simulink model "my_fuzzy"  (Simulink 7.3)
settings: Solver=ode45  StartTime=0.0  StopTime=5000  RelTol=1e-3
values from neighbouring files (symbols this model uses):
  my_fuzzypid =     [fisdata.mat]
libraries: fuzblock x1
settings Model: Creator=sn00632  LastModifiedBy=sn00632
settings SolverCC: MaxConsecutiveMinStep=100  ZeroCrossControl=DisableAll
settings DataIOCC: LimitDataPoints=off
settings DebuggingCC: SolverPrmCheckMsg=none

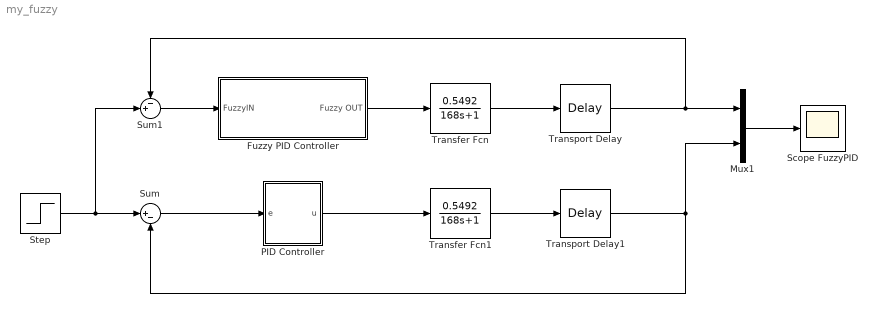
== system my_fuzzy ==
  Fuzzy PID Controller : Subsystem  mask(Fuzzy PID  Controller){my_fuzz=my_fuzzypid}
      mask prompts: my_fuzz "Fis variable:"
      mask help: This a two input and three output fuzzy logic controller
      mask Display: plot(0, -0.3, 6, -0.3, 0, 1.2, 6, 1.2, [0 6], [0 0], [1 2 3],[0 1 0],[2 3 4],[0 1 0],[3 4 5],[0 1 0])
  Mux1 : Mux  Inputs=2
  PID Controller : Subsystem  mask(PID  Controller){P=1.28, I=0.0078, D=5}
      mask prompts: P "Proportional coeff:"; I "Integration  coeff:"; D "Derivatives  coeff:"
      mask help: adjust PID parameters
      mask Display: image(imread('pid_icon.jpg'))
  Scope FuzzyPID : Scope
      settings: SaveName=fuzzout  DataFormat=Array
  Step : Step  Time=10  Before=20  After=60  SampleTime=0
  Sum : Sum  Inputs=|+-  OutDataType=fixdt(1, 16)  OutScaling=2^0
  Sum1 : Sum  Inputs=-+|  OutDataType=fixdt(1, 16)  OutScaling=2^0
  Transfer Fcn : TransferFcn  Numerator=[0.5492]  Denominator=[168 1]
  Transfer Fcn1 : TransferFcn  Numerator=[0.5492]  Denominator=[168 1]
  Transport Delay : TransportDelay  DelayTime=58.5  BufferSize=32768
  Transport Delay1 : TransportDelay  DelayTime=58.5  BufferSize=32768
  wires:
  Step/1 -> Sum/1, Sum1/2
  Sum/1 -> PID Controller/1(e)
  PID Controller/1(u) -> Transfer Fcn1/1
  Transport Delay/1 -> Mux1/1, Sum1/1
  Fuzzy PID Controller/1(Fuzzy OUT) -> Transfer Fcn/1
  Transfer Fcn/1 -> Transport Delay/1
  Transfer Fcn1/1 -> Transport Delay1/1
  Transport Delay1/1 -> Mux1/2, Sum/2
  Mux1/1 -> Scope FuzzyPID/1
  Sum1/1 -> Fuzzy PID Controller/1(" FuzzyIN")

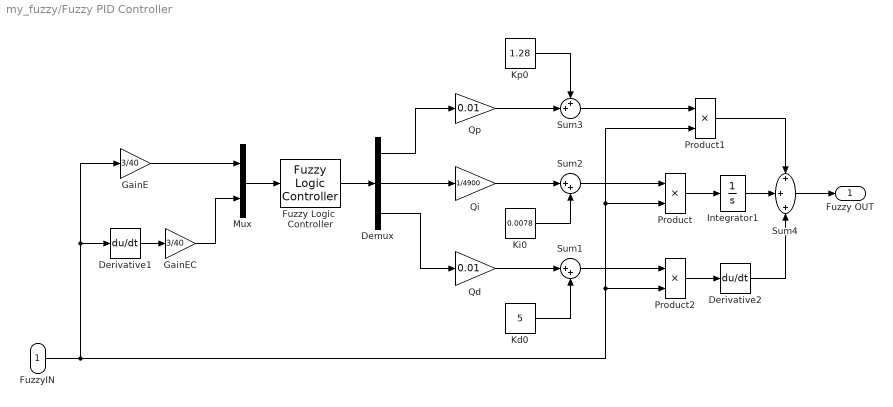
== system my_fuzzy/Fuzzy PID Controller ==
  " FuzzyIN" : Inport
  Demux : Demux  Outputs=3
  Derivative1 : Derivative
  Derivative2 : Derivative
  Fuzzy Logic  Controller : fuzblock/Fuzzy Logic  Controller  SystemSampleTime=-1  fis=my_fuzz
  GainE : Gain  Gain=3/40  ParameterDataType=fixdt(1, 16)  ParameterScaling=2^0  OutDataType=fixdt(1, 16)  OutScaling=2^0
  GainEC : Gain  Gain=3/40  ParameterDataType=fixdt(1, 16)  ParameterScaling=2^0  OutDataType=fixdt(1, 16)  OutScaling=2^0
  Integrator1 : Integrator
  Kd0 : Constant  Value=5  OutDataType=fixdt(1, 16)  OutScaling=2^0
  Ki0 : Constant  Value=0.0078  OutDataType=fixdt(1, 16)  OutScaling=2^0
  Kp0 : Constant  Value=1.28  OutDataType=fixdt(1, 16)  OutScaling=2^0
  Mux : Mux  Inputs=2
  Product : Product  OutDataType=fixdt(1, 16)  OutScaling=2^0  RndMeth=Zero
  Product1 : Product  OutDataType=fixdt(1, 16)  OutScaling=2^0  RndMeth=Zero
  Product2 : Product  OutDataType=fixdt(1, 16)  OutScaling=2^0  RndMeth=Zero
  Qd : Gain  Gain=0.01  ParameterDataType=fixdt(1, 16)  ParameterScaling=2^0  OutDataType=fixdt(1, 16)  OutScaling=2^0
  Qi : Gain  Gain=1/4900  ParameterDataType=fixdt(1, 16)  ParameterScaling=2^0  OutDataType=fixdt(1, 16)  OutScaling=2^0
  Qp : Gain  Gain=0.01  ParameterDataType=fixdt(1, 16)  ParameterScaling=2^0  OutDataType=fixdt(1, 16)  OutScaling=2^0
  Sum1 : Sum  Inputs=|++  OutDataType=fixdt(1, 16)  OutScaling=2^0
  Sum2 : Sum  Inputs=|++  OutDataType=fixdt(1, 16)  OutScaling=2^0
  Sum3 : Sum  Inputs=++|  OutDataType=fixdt(1, 16)  OutScaling=2^0
  Sum4 : Sum  Inputs=+++  OutDataType=fixdt(1, 16)  OutScaling=2^0
  Fuzzy OUT : Outport
  wires:
  Derivative1/1 -> GainEC/1
  GainE/1 -> Mux/1
  GainEC/1 -> Mux/2
  Mux/1 -> Fuzzy Logic  Controller/1
  Fuzzy Logic  Controller/1 -> Demux/1
  Demux/2 -> Qi/1
  Demux/1 -> Qp/1
  Demux/3 -> Qd/1
  Qd/1 -> Sum1/1
  Qi/1 -> Sum2/1
  Product/1 -> Integrator1/1
  Product2/1 -> Derivative2/1
  Product1/1 -> Sum4/1
  Qp/1 -> Sum3/2
  Kp0/1 -> Sum3/1
  Ki0/1 -> Sum2/2
  Kd0/1 -> Sum1/2
  Sum3/1 -> Product1/1
  Sum2/1 -> Product/1
  Sum1/1 -> Product2/1
  Integrator1/1 -> Sum4/2
  Derivative2/1 -> Sum4/3
  " FuzzyIN"/1 -> GainE/1, Derivative1/1, Product2/2, Product/2, Product1/2
  Sum4/1 -> Fuzzy OUT/1

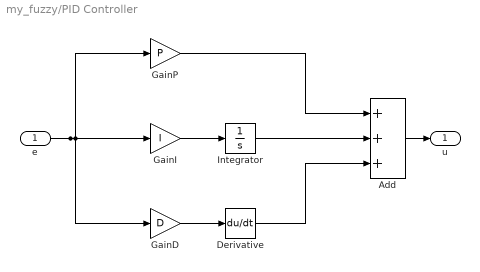
== system my_fuzzy/PID Controller ==
  e : Inport
  Add : Sum  Inputs=+++  OutDataType=fixdt(1, 16)  OutScaling=2^-10
  Derivative : Derivative
  GainD : Gain  Gain=D  ParameterDataType=fixdt(1, 16)  ParameterScaling=2^0  OutDataType=fixdt(1, 16)  OutScaling=2^0
  GainI : Gain  Gain=I  ParameterDataType=fixdt(1, 16)  ParameterScaling=2^0  OutDataType=fixdt(1, 16)  OutScaling=2^0
  GainP : Gain  Gain=P  ParameterDataType=fixdt(1, 16)  ParameterScaling=2^0  OutDataType=fixdt(1, 16)  OutScaling=2^0
  Integrator : Integrator
  u : Outport
  wires:
  Integrator/1 -> Add/2
  Derivative/1 -> Add/3
  GainP/1 -> Add/1
  GainI/1 -> Integrator/1
  GainD/1 -> Derivative/1
  e/1 -> GainD/1, GainI/1, GainP/1
  Add/1 -> u/1
